simulink model "TransposeArchitecture"  (R2014a)
settings: Solver=ode45  StartTime=0.0  StopTime=100  RelTol=1e-3
undefined symbols (not defined in the file): A, N, xlfda_numerator
libraries: xbsIndex_r4 x6, dspsrcs4 x1, JTAGRuntimeCosim_r4 x1
settings Model: Creator=SMDP-C2SD 3  LastModifiedBy=SMDP-C2SD 3

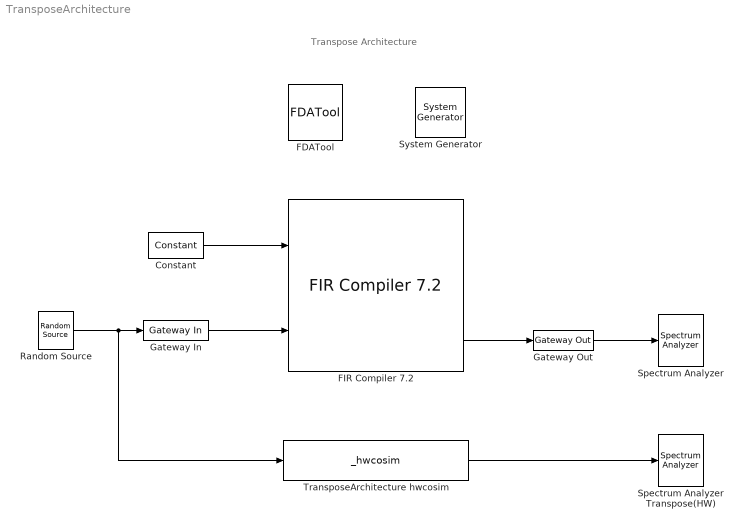
== system TransposeArchitecture ==
  note: Transpose Architecture
  " System Generator" : xbsIndex_r4/ System Generator  Tag=genX  xilinxfamily=zynq  part=xc7z020  speed=-1  package=clg484  synthesis_tool=Vivado  clock_wrapper=Clock Enables  directory=C:/sys_1/hcosim  proj_type=Vivado  Synth_file=Vivado Synthesis Defaults  Impl_file=Vivado Implementation Defaults  testbench=off  simulink_period=1/30  sysclk_period=10  dcm_input_clock_period=10  incr_netlist=off  trim_vbits=Everywhere in SubSystem  dbl_ovrd=According to Block Masks  core_generation=According to Block Masks  run_coregen=off  deprecated_control=off  eval_field=0  block_type=sysgen
  Constant : xbsIndex_r4/Constant  const=1.0  gui_display_data_type=Boolean  arith_type=Boolean  n_bits=16  bin_pt=14  preci_type=Single  exp_width=8  frac_width=24  explicit_period=on  period=1/30  equ=P=C  opselect=C  inp2=PCIN>>17  opr=+  inp1=P  carry=CIN  dbl_ovrd=off  block_type=constant
  FDATool : xbsIndex_r4/FDATool  block_type=fdatool
      settings: infoedit=FDATool
  "FIR Compiler 7.2 " : xbsIndex_r4/FIR Compiler 7.2   coefficientvector=xlfda_numerator('FDATool')  coefficient_sets=1  coefficient_reload=off  filter_type=Single_Rate  rate_change_type=Integer  interpolation_rate=1  decimation_rate=1  zero_pack_factor=1  channel_sequence=Basic  number_channels=1  pattern_list='P4-0,P4-1,P4-2,P4-3,P4-4'  number_paths=1  ratespecification=Output_Sample_Period  sampleperiod=1  hardwareoversamplingrate=1  coefficient_sign=Signed  quantization=Quantize_Only  coefficient_width=16  bestprecision=off  coefficient_fractional_bits=14  coefficient_structure=Non_Symmetric  output_rounding_mode=Full_Precision  output_width=32  filter_architecture=Transpose_Multiply_Accumulate  optimization_goal=Area  optimization_list='None'  data_buffer_type=Automatic  coefficient_buffer_type=Automatic  input_buffer_type=Automatic  output_buffer_type=Automatic  preference_for_other_storage=Automatic  multi_column_support=Automatic  columnconfig='20,20,60,60,6'  inter_column_pipe_length=4  data_has_tlast=Not_Required  m_data_has_tready=off  s_data_has_fifo=off  s_data_has_tuser=Not_Required  m_data_has_tuser=Not_Required  s_config_sync_mode=On_Vector  s_config_method=Single  num_reload_slots=1  has_aclken=off  has_aresetn=off  infoeditControl=ARESETn must be asserted for a minimum of 2 cycles  reset_data_vector=on  trim_axipin_name=on  simulation_type=hybrid_sim  simulation_model=sysgen:xfirv7_2_cmodel  data_path_portlist={ 's_axis_data_tdata', 'm_axis_data_tdata' }  passband_min=0.0  passband_max=0.5  stopband_min=0.5  stopband_max=1.0  filter_selection=1  gui_behaviour='Sysgen_GUI'  data_sign=Signed  data_width=16  data_fractional_bits=0  data_tuser_width=1  wrapper_available=true  ip_wrap_arbitrary_binary_point=true  ip_name=FIR Compiler  ip_version=7.2  dsptool_ready=true  ipcore_usecache=true  ipcore_useipmodelcache=true  port_translation_map={ 'aclken' => 'en', 'aresetn' => 'rst' }  run_core_at_system_period=true  ipcore_xco_need_fpga_part=true  block_type=fir_compiler_v7_2
      settings: infoedit=Maximum Possible : Maximizes oversampling rate. Abstracted input handshake (no s_data_tvalid) and automatic rate propagation.<br>Hardware Oversampling Rate : Specifies oversampling rate relative to the input sample period. Abstracted input handshake (no s_data_tvalid) and automatic rate propagation.<br>Input/Output Sample Period : Specifies absolute oversampling rate. No input handshake abstraction (exposes s_data_tvalid) and no rate propagation.
  Gateway In : xbsIndex_r4/Gateway In  gui_display_data_type=Fixed-point  arith_type="Signed  (2's comp)"  n_bits=8  bin_pt=6  preci_type=Single  exp_width=8  frac_width=24  rows=1  columns=1  quantization="Round  (unbiased: +/- Inf)"  overflow=Saturate  period=1/30  UseAsADC=off  ADCChannel='1'  interface=None  automatic_assignment=on  address_offset=hex2dec('00')  intf_name=''  intf_description=''  timing_constraint=None  locs_specified=off  LOCs={}  io_standard={}  inherit_from_input=off  hdl_port=on  dbl_ovrd=off  block_type=gatewayin
  Gateway Out : xbsIndex_r4/Gateway Out  inherit_from_input=off  hdl_port=on  rows=1  columns=1  UseAsDAC=off  DACChannel='1'  interface=None  automatic_assignment=on  address_offset=hex2dec('00')  intf_name=''  intf_description=''  timing_constraint=None  locs_specified=off  LOCs={}  io_standard={}  block_type=gatewayout
  Random Source : dspsrcs4/Random Source  SrcType=Gaussian  NormMethod=Ziggurat  CltLength=12  MinVal=0  MaxVal=1  MeanVal=0  VarVal=1  RepMode=Not repeatable  rawSeed=1  IsInherit=off  SampMode=Discrete  SampTime=1/30  SampFrame=1  DataType=Double  OutComplex=Real
  Spectrum Analyzer : SpectrumAnalyzer
  Spectrum Analyzer Transpose(HW) : SpectrumAnalyzer
  TransposeArchitecture hwcosim : JTAGRuntimeCosim_r4/_hwcosim  clkSrc=Single Stepped  hasCombinationalPath=on  bitfileName=C:\sys_1\hcosim\transposearchitecture.bit  skipConfig=off  dispPartInfo=off  useZynqReconfigScript=off  cable=Auto Detect  speed=N/A  cablePort=N/A  cableLocation=Local  shareCable=off  design_xtable=|  engineDll=JTAGCosimEngine.dll  cableWaitTime=10  bscanPos=-1  IRLengths=[]  useWaitBox=1  hasBufgmux=on  Scheme=Cosim  useCmdProc=1  hasProc=0  useImpact=0  printLogFile=0  userChain=2  block_type=jtagcosim
      | {
      |     'clkWrapper' => 'transposearchitecture',
      |     'burstMode' => false,
      |     'burstFifoDepth' => '1024',
      |     'shared_memories' => {},
      |     'clocksGcd' => 1,
      |     'device' => {
      |       'family' => 'zynq',
      |       'part' => 'xc7z020',
      |       'package' => 'clg484',
      |       'speed' => -1,
      |     },
      |     'ports' => {
      |       'gateway_in' => {
      |         'direction' => 'in',
      |         'width' => 8,
      |         'name' => 'gateway_in',
      |         'period' => 1,
      |         'icon_text' => 'Gateway In',
      |         'type' => 'Fix_8_6',
      |         'arithmetic_type' => 'xlSigned',
      |         'dat_file' => 'transposearchitecture_gateway_in.dat',
      |         'bin_pt' => 6,
      |         'addr_offset' => 0,
      |         'bd_port_index' => 0,
      |       },
      |       'gateway_out' => {
      |         'direction' => 'out',
      |         'width' => 24,
      |         'name' => 'gateway_out',
      |         'period' => 1,
      |         'icon_text' => 'Gateway Out',
      |         'type' => 'Fix_24_20',
      |         'arithmetic_type' => 'xlSigned',
      |         'dat_file' => 'transposearchitecture_gateway_out.dat',
      |         'bin_pt' => 20,
      |         'addr_offset' => 4,
      |         'bd_port_index' => 0,
      |       },
      |     },
      |   }
  wires:
  Constant/1 -> "FIR Compiler 7.2 "/1
  Gateway In/1 -> "FIR Compiler 7.2 "/2
  "FIR Compiler 7.2 "/3 -> Gateway Out/1
  Gateway Out/1 -> Spectrum Analyzer/1
  Random Source/1 -> TransposeArchitecture hwcosim/1, Gateway In/1
  TransposeArchitecture hwcosim/1 -> Spectrum Analyzer Transpose(HW)/1
